simulink model "viterbi_check"  (Simulink 7.9)
settings: Solver=ode45  StartTime=0.0  StopTime=10  RelTol=1e-3
libraries: commcnvcod2 x2, commrandsrc2 x1, commsink2 x1
settings Model: Creator=ArunKB  LastModifiedBy=ArunKB

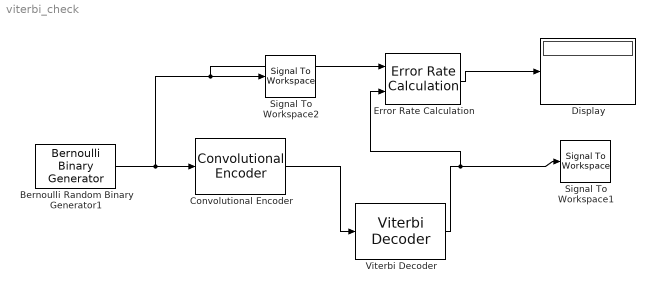
== system viterbi_check ==
  Bernoulli Random Binary Generator1 : commrandsrc2/Bernoulli Binary Generator  P=0.5  seed=241  Ts=.001  frameBased=on  sampPerFrame=45  orient=off  outDataType=double
  Convolutional Encoder : commcnvcod2/Convolutional Encoder  trellis=poly2trellis(7, [171 133])  opMode=Truncated (reset every frame)  DelayedResetAction=off  hasIniStPort=off  hasFinStPort=off  usePuncVector=off  punctureVector=[1; 1; 0; 1; 0; 1]  reset=Unused parameter value
  Display : Display
  Error Rate Calculation : commsink2/Error Rate Calculation  N=0  st_delay=0  cp_mode=Entire frame  subframe=[]  PMode=Port  WsName=ErrorVec  RsMode2=off  stop=off  numErr=100  maxBits=1e6
  Signal To Workspace1 : SignalToWorkspace  VariableName=output
      settings: CopyFcn=dspblkcopystw(gcbh);
  Signal To Workspace2 : SignalToWorkspace  VariableName=input
      settings: CopyFcn=dspblkcopystw(gcbh);
  Viterbi Decoder : commcnvcod2/Viterbi Decoder  trellis=poly2trellis(7, [171 133])  isPunctured=off  punctureVector=[1; 1; 0; 1; 0; 1]  erasures=off  dectype=Hard decision  runSigValErrCheck=off  nsdecb=2  smWordLength=16  tbdepth=45  opmode=Truncated  reset=off  outDataType=Inherit via internal rule  delayedResetAction=off
  wires:
  Bernoulli Random Binary Generator1/1 -> Convolutional Encoder/1, Signal To Workspace2/1, Error Rate Calculation/1
  Convolutional Encoder/1 -> Viterbi Decoder/1
  Viterbi Decoder/1 -> Signal To Workspace1/1, Error Rate Calculation/2
  Error Rate Calculation/1 -> Display/1
